simulink model "Book423"  (R2019b)
settings: Solver=ode4  StartTime=0.001  StopTime=20  FixedStep=0.001  RelTol=1e-3
settings Model: Creator=xyh  LastModifiedBy=xyh

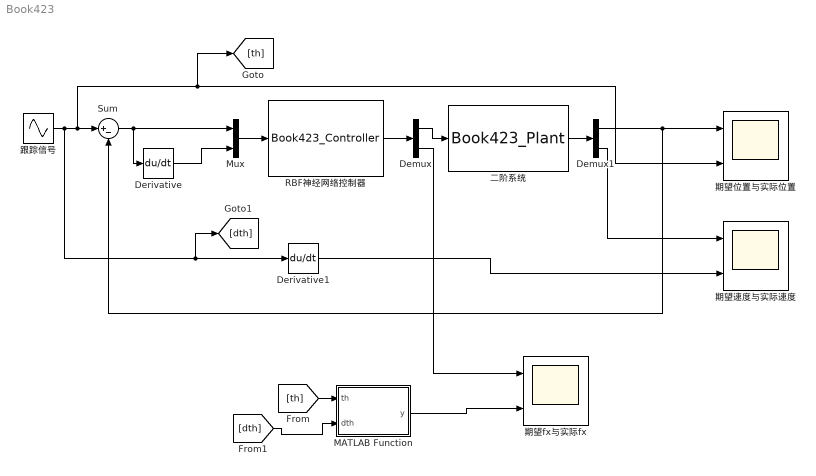
== system Book423 ==
  Demux : Demux  Outputs=2
  Demux1 : Demux  Outputs=2
  Derivative : Derivative
  Derivative1 : Derivative
  MATLAB Function : MATLAB Function  TreatAsAtomicUnit=on
  Mux : Mux  Inputs=2
  RBF神经网络控制器 : S-Function  FunctionName=Book423_Controller  SFunctionDeploymentMode=off  EnableBusSupport=off
  Sum : Sum  Inputs=|+-
  二阶系统 : S-Function  FunctionName=Book423_Plant  SFunctionDeploymentMode=off  EnableBusSupport=off
  期望fx与实际fx : Scope  NumInputPorts=2
  期望位置与实际位置 : Scope  NumInputPorts=2
  期望速度与实际速度 : Scope  NumInputPorts=2
  跟踪信号 : Sin  SampleTime=0
  wires:
  MATLAB Function/1(y) -> 期望fx与实际fx/2
  [dth] -> MATLAB Function/2(dth)
  [th] -> MATLAB Function/1(th)
  Demux/2 -> 期望fx与实际fx/1
  Derivative1/1 -> 期望速度与实际速度/2
  Mux/1 -> RBF神经网络控制器/1
  跟踪信号/1 -> [dth], Derivative1/1, [th], 期望位置与实际位置/2, Sum/1
  Demux1/1 -> 期望位置与实际位置/1, Sum/2
  Demux1/2 -> 期望速度与实际速度/1
  RBF神经网络控制器/1 -> Demux/1
  二阶系统/1 -> Demux1/1
  Derivative/1 -> Mux/2
  Sum/1 -> Derivative/1, Mux/1
  Demux/1 -> 二阶系统/1

== matlab function Book423/MATLAB Function ==
  data: th input; y output; dth input
function y = fcn(th, dth)
%#codegen
f = -25 * dth - 10 * th;
y = f;
